simulink model "SimulinkBolaPrato"  (R2020a)
settings: Solver=VariableStepAuto  StartTime=0.0  StopTime=inf  RelTol=1e-3
values from neighbouring files (symbols this model uses):
  A = [0 1;0 -fc/(J/Raio^2+m)]    [TCCMATLAB.m]
  B = [0;-m*g*d/(L*(J/Raio^2+m))]    [TCCMATLAB.m]
  C = [1 0]    [TCCMATLAB.m]
  d = 0.03    [TCCMATLAB.m]
  Kbar = Nu + Klqr*Nx    [TCCMATLAB.m]
  Ki = -K(3)    [TCCMATLAB.m]
  Klqr = lqr(A,B,Q,R)    [TCCMATLAB.m]
  Kt = [K(1) K(2)]    [TCCMATLAB.m]
  L = 1.3    [TCCMATLAB.m]
  Raio = 0.05    [TCCMATLAB.m]
  x0 = 0    [TCCMATLAB.m]
libraries: vrlib x7
settings Model: EnablePacing=on  Creator=Diego  LastModifiedBy=Diego

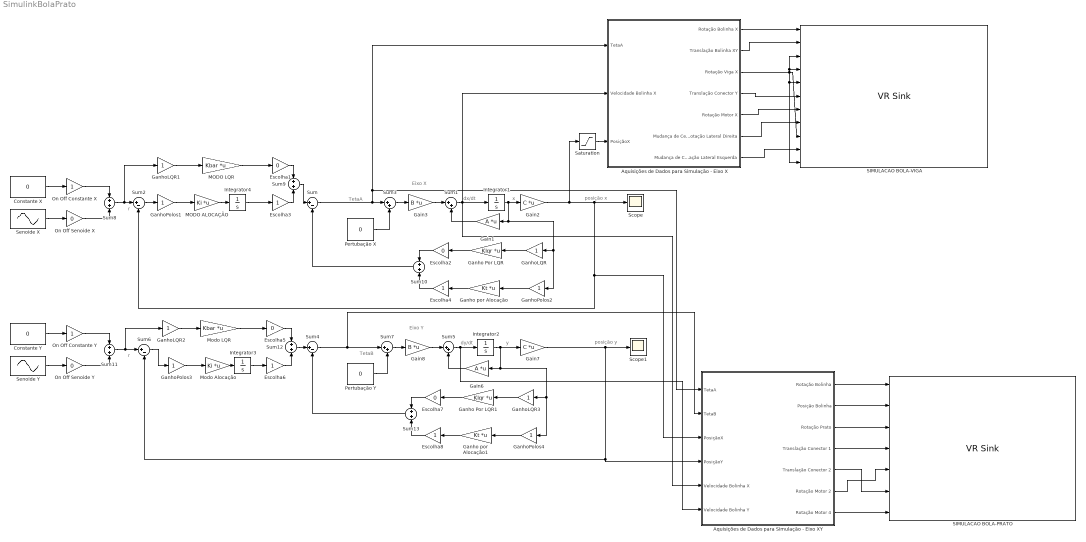
== system SimulinkBolaPrato ==
  note: r
  note: x
  note: posição x
  note: dx/dt
  note: TetaA
  note: Eixo X
  note: TetaB
  note: posição y
  note: dy/dt
  note: y
  note: Eixo Y
  note: r
  Aquisições de Dados para Simulação - Eixo X : Subsystem
  Aquisições de Dados para Simulação - Eixo XY : Subsystem
  Constante X : Constant  Value=0
  Constante Y : Constant  Value=0
  Escolha{1..2,5,7} (4 alike) : Gain  Gain=0
  Escolha{3..4,6,8} (4 alike) : Gain
  Gain1 : Gain  Gain=A  Multiplication=Matrix(K*u)
  Gain2 : Gain  Gain=C  Multiplication=Matrix(K*u)
  Gain3 : Gain  Gain=B  Multiplication=Matrix(K*u)
  Gain6 : Gain  Gain=A  Multiplication=Matrix(K*u)
  Gain7 : Gain  Gain=C  Multiplication=Matrix(K*u)
  Gain8 : Gain  Gain=B  Multiplication=Matrix(K*u)
  Ganho Por LQR : Gain  Gain=Klqr  Multiplication=Matrix(K*u)
  Ganho Por LQR1 : Gain  Gain=Klqr  Multiplication=Matrix(K*u)
  Ganho por Alocação : Gain  Gain=Kt  Multiplication=Matrix(K*u)
  Ganho por Alocação1 : Gain  Gain=Kt  Multiplication=Matrix(K*u)
  GanhoLQR{,1..3} (4 alike) : Gain
  GanhoPolos{1..4} (4 alike) : Gain
  Integrator1 : Integrator  InitialCondition=x0
  Integrator2 : Integrator  InitialCondition=x0
  Integrator3 : Integrator  InitialCondition=x0  AbsoluteTolerance=1
  Integrator4 : Integrator  InitialCondition=x0  AbsoluteTolerance=1
  MODO ALOCAÇÃO : Gain  Gain=Ki  Multiplication=Matrix(K*u)
  MODO LQR : Gain  Gain=Kbar  Multiplication=Matrix(K*u)
  Modo Alocação : Gain  Gain=Ki  Multiplication=Matrix(K*u)
  Modo LQR : Gain  Gain=Kbar  Multiplication=Matrix(K*u)
  On Off Constante X : Gain
  On Off Constante Y : Gain
  On Off Senoide X : Gain  Gain=0
  On Off Senoide Y : Gain  Gain=0
  Pertubação X : Constant  Value=0
  Pertubação Y : Constant  Value=0
  SIMULACAO BOLA-PRATO : vrlib/VR Sink  InstantiateOnLoad=on  SampleTime=-1  ViewEnable=on  RemoteChange=off  RemoteView=off  FieldsWritten=Ball.rotation.4.1.1.double#Ball.translation.3.1.1.double#BaseViga.rotation.4.1.1.double#Conector.translation.3.1.1.double#Motor2.rotation.4.1.1.double#Conector2.translation.3.1.1.double#Motor4.rotation.4.1.1.double  WorldFileName=Ball&Plate.x3d  WorldDescription=Simulação Bola-Prato  AutoView=off  VideoDimensions=[]  AllowVariableSize=off
  SIMULACAO BOLA-VIGA : vrlib/VR Sink  InstantiateOnLoad=on  SampleTime=0.01  ViewEnable=on  RemoteChange=off  RemoteView=off  FieldsWritten=Ball.rotation.4.1.1.double#Ball.translation.3.1.1.double#BaseViga.rotation.4.1.1.double#LadoTraseiroViga.rotation.4.1.1.double#LadoFrontalViga.rotation.4.1.1.double#Conector.translation.3.1.1.double#Motor2.rotation.4.1.1.double#LadoDireitoViga.center.3.1.1.double#LadoDireitoViga.rotation.4.1.1.double#LadoEsquerdoViga.center.3.1.1.double#LadoEsquerdoViga.rotation.4.1.1.double  WorldFileName=Ball&Beam.x3d  AutoView=off  VideoDimensions=[]  AllowVariableSize=off
  Saturation : Saturate  UpperLimit=0.59  LowerLimit=-0.59
  Scope : Scope
  Scope1 : Scope
  Senoide X : Sin  Amplitude=0  SampleTime=0
  Senoide Y : Sin  Amplitude=0  SampleTime=0
  Sum{,2,4,6} (4 alike) : Sum  Inputs=|+-
  Sum{1,3,5,7} (4 alike) : Sum  Inputs=|++
  Sum{8..13} (6 alike) : Sum  Inputs=+|+
  wires:
  Gain3/1 -> Sum1/1
  Gain1/1 -> Sum1/2
  Sum3/1 -> Gain3/1
  MODO ALOCAÇÃO/1 -> Integrator4/1
  Ganho por Alocação/1 -> Escolha4/1
  Sum10/1 -> Sum/2
  Ganho Por LQR/1 -> Escolha2/1
  Senoide X/1 -> On Off Senoide X/1
  Integrator4/1 -> Escolha3/1
  Sum9/1 -> Sum/1
  MODO LQR/1 -> Escolha1/1
  Gain6/1 -> Sum5/2
  Gain8/1 -> Sum5/1
  Sum5/1 -> Aquisições de Dados para Simulação - Eixo XY/6(Velocidade Bolinha Y), Integrator2/1
  Sum7/1 -> Gain8/1
  Integrator2/1 -> GanhoPolos4/1, GanhoLQR3/1, Gain6/1, Gain7/1
  Sum11/1 -> GanhoLQR2/1, Sum6/1
  Gain7/1 -> Sum6/2, Aquisições de Dados para Simulação - Eixo XY/4(PosiçãoY), Scope1/1
  Integrator1/1 -> Gain2/1, GanhoPolos2/1, GanhoLQR/1, Gain1/1
  Gain2/1 -> Saturation/1, Aquisições de Dados para Simulação - Eixo XY/3(PosiçãoX), Sum2/2, Scope/1
  Sum1/1 -> Aquisições de Dados para Simulação - Eixo XY/5(Velocidade Bolinha X), Aquisições de Dados para Simulação - Eixo X/2(Velocidade Bolinha X), Integrator1/1
  Aquisições de Dados para Simulação - Eixo X/1(Rotação Bolinha X) -> SIMULACAO BOLA-VIGA/1
  Aquisições de Dados para Simulação - Eixo X/3(Rotação Viga X) -> SIMULACAO BOLA-VIGA/11, SIMULACAO BOLA-VIGA/5, SIMULACAO BOLA-VIGA/3, SIMULACAO BOLA-VIGA/4, SIMULACAO BOLA-VIGA/9
  Aquisições de Dados para Simulação - Eixo X/2(Translação Bolinha XY) -> SIMULACAO BOLA-VIGA/2
  Aquisições de Dados para Simulação - Eixo X/7(Mudança de Centro de Rotação Lateral Esquerda) -> SIMULACAO BOLA-VIGA/10
  Aquisições de Dados para Simulação - Eixo X/6(Mudança de Centro de Rotação Lateral Direita) -> SIMULACAO BOLA-VIGA/8
  Aquisições de Dados para Simulação - Eixo X/5(Rotação Motor X) -> SIMULACAO BOLA-VIGA/7
  Aquisições de Dados para Simulação - Eixo X/4(Translação Conector Y) -> SIMULACAO BOLA-VIGA/6
  Sum4/1 -> Sum7/1, Aquisições de Dados para Simulação - Eixo XY/2(TetaB)
  Sum/1 -> Aquisições de Dados para Simulação - Eixo XY/1(TetaA), Aquisições de Dados para Simulação - Eixo X/1(TetaA), Sum3/1
  Constante X/1 -> On Off Constante X/1
  Aquisições de Dados para Simulação - Eixo XY/1(Rotação Bolinha) -> SIMULACAO BOLA-PRATO/1
  Aquisições de Dados para Simulação - Eixo XY/2(Posição Bolinha) -> SIMULACAO BOLA-PRATO/2
  Aquisições de Dados para Simulação - Eixo XY/3(Rotação Prato) -> SIMULACAO BOLA-PRATO/3
  Aquisições de Dados para Simulação - Eixo XY/4(Translação Conector 1) -> SIMULACAO BOLA-PRATO/4
  Aquisições de Dados para Simulação - Eixo XY/6(Rotação Motor 2) -> SIMULACAO BOLA-PRATO/5
  Aquisições de Dados para Simulação - Eixo XY/5(Translação Conector 2) -> SIMULACAO BOLA-PRATO/6
  Aquisições de Dados para Simulação - Eixo XY/7(Rotação Motor 4) -> SIMULACAO BOLA-PRATO/7
  Saturation/1 -> Aquisições de Dados para Simulação - Eixo X/3(PosiçãoX)
  Sum8/1 -> GanhoLQR1/1, Sum2/1
  On Off Constante X/1 -> Sum8/1
  On Off Senoide X/1 -> Sum8/2
  Pertubação X/1 -> Sum3/2
  Escolha1/1 -> Sum9/1
  Escolha3/1 -> Sum9/2
  Escolha2/1 -> Sum10/1
  Escolha4/1 -> Sum10/2
  GanhoLQR1/1 -> MODO LQR/1
  GanhoPolos1/1 -> MODO ALOCAÇÃO/1
  Sum2/1 -> GanhoPolos1/1
  GanhoPolos2/1 -> Ganho por Alocação/1
  GanhoLQR/1 -> Ganho Por LQR/1
  Constante Y/1 -> On Off Constante Y/1
  On Off Senoide Y/1 -> Sum11/2
  On Off Constante Y/1 -> Sum11/1
  Modo LQR/1 -> Escolha5/1
  Modo Alocação/1 -> Integrator3/1
  GanhoPolos3/1 -> Modo Alocação/1
  Integrator3/1 -> Escolha6/1
  GanhoLQR2/1 -> Modo LQR/1
  Escolha6/1 -> Sum12/2
  Escolha5/1 -> Sum12/1
  Sum12/1 -> Sum4/1
  Sum6/1 -> GanhoPolos3/1
  Ganho Por LQR1/1 -> Escolha7/1
  Sum13/1 -> Sum4/2
  Ganho por Alocação1/1 -> Escolha8/1
  Escolha7/1 -> Sum13/1
  Escolha8/1 -> Sum13/2
  GanhoLQR3/1 -> Ganho Por LQR1/1
  GanhoPolos4/1 -> Ganho por Alocação1/1
  Pertubação Y/1 -> Sum7/2
  Senoide Y/1 -> On Off Senoide Y/1

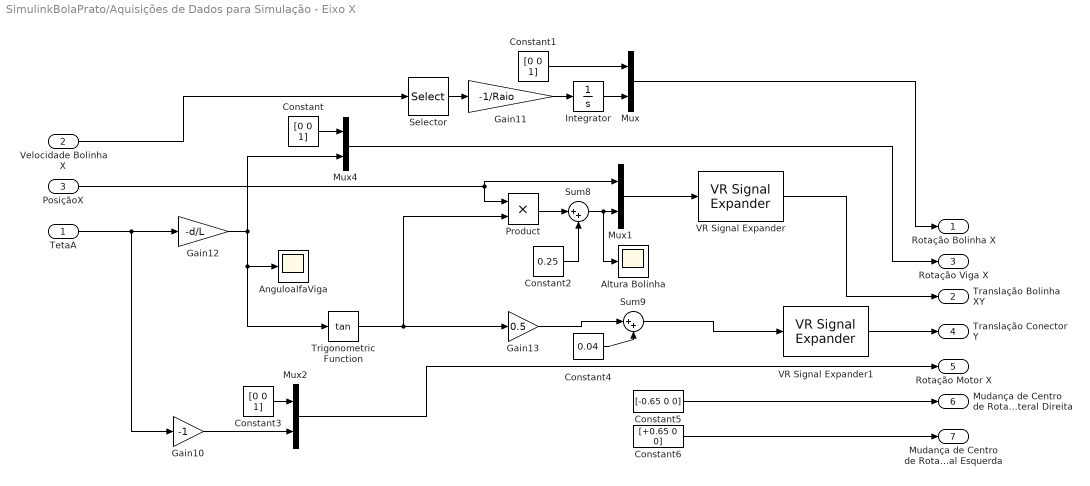
== system SimulinkBolaPrato/Aquisições de Dados para Simulação - Eixo X ==
  TetaA : Inport
  Velocidade Bolinha X : Inport  Port=2
  PosiçãoX : Inport  Port=3
  Altura Bolinha : Scope
  AnguloalfaViga : Scope
  Constant : Constant  Value=[0 0 1]
  Constant1 : Constant  Value=[0 0 1]
  Constant2 : Constant  Value=0.25
  Constant3 : Constant  Value=[0 0 1]
  Constant4 : Constant  Value=0.04
  Constant5 : Constant  Value=[-0.65 0 0]
  Constant6 : Constant  Value=[+0.65 0 0]
  Gain10 : Gain  Gain=-1
  Gain11 : Gain  Gain=-1/Raio
  Gain12 : Gain  Gain=-d/L
  Gain13 : Gain  Gain=0.5
  Integrator : Integrator
  Mux{,1..2,4} (4 alike) : Mux  Inputs=2
  Product : Product
  Selector : Selector  InputPortWidth=2  IndexOptions=Index vector (dialog)  Indices=[1]  OutputSizes=1
  Sum8 : Sum  Inputs=|++
  Sum9 : Sum  Inputs=|++
  Trigonometric Function : Trigonometry  Operator=tan
  VR Signal Expander : vrlib/VR Signal Expander  outwidth=3  outidx=[1 2]
  VR Signal Expander1 : vrlib/VR Signal Expander  outwidth=3  outidx=[2]
  Rotação Bolinha X : Outport
  Translação Bolinha XY : Outport  Port=2
  Rotação Viga X : Outport  Port=3
  Translação Conector Y : Outport  Port=4
  Rotação Motor X : Outport  Port=5
  Mudança de Centro de Rotação Lateral Direita : Outport  Port=6
  Mudança de Centro de Rotação Lateral Esquerda : Outport  Port=7
  wires:
  Constant3/1 -> Mux2/1
  Sum8/1 -> Altura Bolinha/1, Mux1/2
  PosiçãoX/1 -> Product/1, Mux1/1
  Gain13/1 -> Sum9/1
  Sum9/1 -> VR Signal Expander1/1
  Gain10/1 -> Mux2/2
  Constant4/1 -> Sum9/2
  Product/1 -> Sum8/1
  Trigonometric Function/1 -> Product/2, Gain13/1
  Gain12/1 -> Trigonometric Function/1, AnguloalfaViga/1, Mux4/2
  VR Signal Expander1/1 -> Translação Conector Y/1
  TetaA/1 -> Gain10/1, Gain12/1
  Constant2/1 -> Sum8/2
  Constant/1 -> Mux4/1
  Mux1/1 -> VR Signal Expander/1
  Mux2/1 -> Rotação Motor X/1
  Constant5/1 -> Mudança de Centro de Rotação Lateral Direita/1
  Mux4/1 -> Rotação Viga X/1
  Constant6/1 -> Mudança de Centro de Rotação Lateral Esquerda/1
  VR Signal Expander/1 -> Translação Bolinha XY/1
  Velocidade Bolinha X/1 -> Selector/1
  Constant1/1 -> Mux/1
  Gain11/1 -> Integrator/1
  Selector/1 -> Gain11/1
  Mux/1 -> Rotação Bolinha X/1
  Integrator/1 -> Mux/2

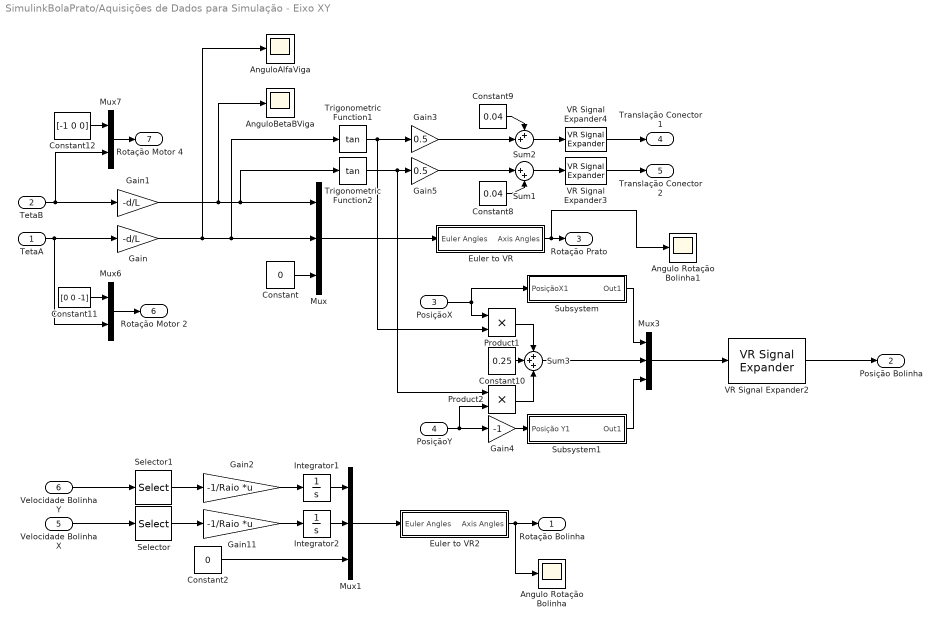
== system SimulinkBolaPrato/Aquisições de Dados para Simulação - Eixo XY ==
  TetaA : Inport
  TetaB : Inport  Port=2
  PosiçãoX : Inport  Port=3
  PosiçãoY : Inport  Port=4
  Velocidade Bolinha X : Inport  Port=5
  Velocidade Bolinha Y : Inport  Port=6
  Angulo Rotação Bolinha : Scope
  Angulo Rotação Bolinha1 : Scope
  AnguloAlfaViga : Scope
  AnguloBetaBViga : Scope
  Constant : Constant  Value=0
  Constant10 : Constant  Value=0.25
  Constant11 : Constant  Value=[0 0 -1]
  Constant12 : Constant  Value=[-1 0 0]
  Constant2 : Constant  Value=0
  Constant8 : Constant  Value=0.04
  Constant9 : Constant  Value=0.04
  Euler to VR : Subsystem
  Euler to VR2 : Subsystem
  Gain : Gain  Gain=-d/L
  Gain1 : Gain  Gain=-d/L
  Gain11 : Gain  Gain=-1/Raio  Multiplication=Matrix(K*u)
  Gain2 : Gain  Gain=-1/Raio  Multiplication=Matrix(K*u)
  Gain3 : Gain  Gain=0.5
  Gain4 : Gain  Gain=-1
  Gain5 : Gain  Gain=0.5
  Integrator1 : Integrator
  Integrator2 : Integrator
  Mux : Mux  Inputs=3
  Mux1 : Mux  Inputs=3
  Mux3 : Mux  Inputs=3
  Mux6 : Mux  Inputs=2
  Mux7 : Mux  Inputs=2
  Product1 : Product
  Product2 : Product
  Selector : Selector  InputPortWidth=2  IndexOptions=Index vector (dialog)  Indices=[1]  OutputSizes=1
  Selector1 : Selector  InputPortWidth=2  IndexOptions=Index vector (dialog)  Indices=[1]  OutputSizes=1
  Subsystem : Subsystem
  Subsystem1 : Subsystem
  Sum1 : Sum  Inputs=|++
  Sum2 : Sum  Inputs=++|
  Sum3 : Sum  Inputs=+++
  Trigonometric Function1 : Trigonometry  Operator=tan
  Trigonometric Function2 : Trigonometry  Operator=tan
  VR Signal Expander2 : vrlib/VR Signal Expander  outwidth=3  outidx=[1 2 3]
  VR Signal Expander3 : vrlib/VR Signal Expander  outwidth=3  outidx=[2]
  VR Signal Expander4 : vrlib/VR Signal Expander  outwidth=3  outidx=[2]
  Rotação Bolinha : Outport
  Posição Bolinha : Outport  Port=2
  Rotação Prato : Outport  Port=3
  Translação Conector 1 : Outport  Port=4
  Translação Conector 2 : Outport  Port=5
  Rotação Motor 2 : Outport  Port=6
  Rotação Motor 4 : Outport  Port=7
  wires:
  Mux/1 -> Euler to VR/1(Euler Angles)
  Constant/1 -> Mux/3
  Gain/1 -> AnguloAlfaViga/1, Trigonometric Function1/1, Mux/2
  Gain1/1 -> AnguloBetaBViga/1, Mux/1, Trigonometric Function2/1
  TetaB/1 -> Gain1/1, Mux7/2
  Mux3/1 -> VR Signal Expander2/1
  Selector1/1 -> Gain2/1
  Velocidade Bolinha Y/1 -> Selector1/1
  Mux1/1 -> Euler to VR2/1(Euler Angles)
  Constant2/1 -> Mux1/3
  PosiçãoY/1 -> Product2/2, Gain4/1
  VR Signal Expander2/1 -> Posição Bolinha/1
  Euler to VR/1(Axis Angles) -> Angulo Rotação Bolinha1/1, Rotação Prato/1
  Trigonometric Function1/1 -> Product1/2, Gain3/1
  Trigonometric Function2/1 -> Product2/1, Gain5/1
  VR Signal Expander3/1 -> Translação Conector 2/1
  Constant8/1 -> Sum1/2
  Sum1/1 -> VR Signal Expander3/1
  Gain5/1 -> Sum1/1
  VR Signal Expander4/1 -> Translação Conector 1/1
  Sum2/1 -> VR Signal Expander4/1
  Gain3/1 -> Sum2/2
  Constant9/1 -> Sum2/1
  Selector/1 -> Gain11/1
  Velocidade Bolinha X/1 -> Selector/1
  Product1/1 -> Sum3/1
  Product2/1 -> Sum3/3
  Constant10/1 -> Sum3/2
  Sum3/1 -> Mux3/2
  TetaA/1 -> Gain/1, Mux6/2
  Constant11/1 -> Mux6/1
  Mux6/1 -> Rotação Motor 2/1
  Mux7/1 -> Rotação Motor 4/1
  Constant12/1 -> Mux7/1
  PosiçãoX/1 -> Subsystem/1(PosiçãoX1), Product1/1
  Subsystem/1(Out1) -> Mux3/1
  Gain4/1 -> Subsystem1/1(Posição Y1)
  Subsystem1/1(Out1) -> Mux3/3
  Gain2/1 -> Integrator1/1
  Gain11/1 -> Integrator2/1
  Euler to VR2/1(Axis Angles) -> Rotação Bolinha/1, Angulo Rotação Bolinha/1
  Integrator1/1 -> Mux1/1
  Integrator2/1 -> Mux1/2

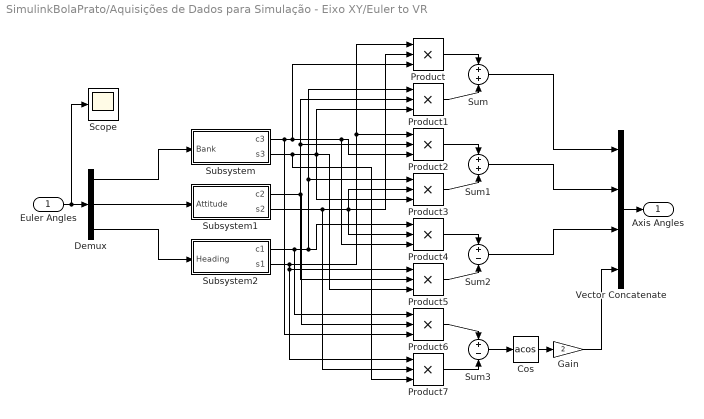
== system SimulinkBolaPrato/Aquisições de Dados para Simulação - Eixo XY/Euler to VR ==
  Euler Angles : Inport
  Cos : Trigonometry  Operator=acos
  Demux : Demux  Outputs=3
      settings: DisplayOption=none
  Gain : Gain  Gain=2
  Product{,1..7} (8 alike) : Product  Inputs=3
  Scope : Scope
  Subsystem : Subsystem
  Subsystem1 : Subsystem
  Subsystem2 : Subsystem
  Sum : Sum  Inputs=+|+
  Sum1 : Sum  Inputs=+|+
  Sum2 : Sum  Inputs=+|-
  Sum3 : Sum  Inputs=+|-
  Vector Concatenate : Concatenate  NumInputs=4
  Axis Angles : Outport
  wires:
  Euler Angles/1 -> Scope/1, Demux/1
  Demux/1 -> Subsystem/1(Bank)
  Demux/3 -> Subsystem2/1(Heading)
  Demux/2 -> Subsystem1/1(Attitude)
  Subsystem2/2(s1) -> Product7/1, Product5/1, Product2/1, Product/1
  Subsystem1/2(s2) -> Product7/2, Product3/2, Product/2, Product4/2
  Subsystem/1(c3) -> Product6/3, Product4/3, Product2/3, Product/3
  Subsystem2/1(c1) -> Product6/1, Product4/1, Product3/1, Product1/1
  Subsystem1/1(c2) -> Product6/2, Product5/2, Product2/2, Product1/2
  Subsystem/2(s3) -> Product7/3, Product5/3, Product1/3, Product3/3
  Product/1 -> Sum/1
  Product1/1 -> Sum/2
  Product2/1 -> Sum1/1
  Product3/1 -> Sum1/2
  Product4/1 -> Sum2/1
  Product5/1 -> Sum2/2
  Product6/1 -> Sum3/1
  Product7/1 -> Sum3/2
  Sum3/1 -> Cos/1
  Cos/1 -> Gain/1
  Gain/1 -> Vector Concatenate/4
  Sum/1 -> Vector Concatenate/1
  Sum1/1 -> Vector Concatenate/2
  Sum2/1 -> Vector Concatenate/3
  Vector Concatenate/1 -> Axis Angles/1

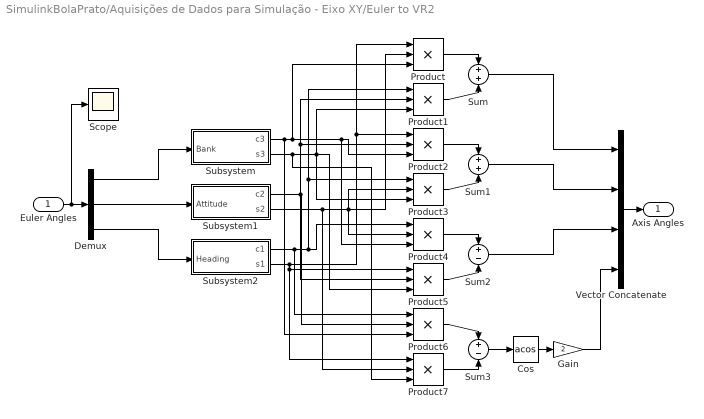
== system SimulinkBolaPrato/Aquisições de Dados para Simulação - Eixo XY/Euler to VR2 ==
  Euler Angles : Inport
  Cos : Trigonometry  Operator=acos
  Demux : Demux  Outputs=3
      settings: DisplayOption=none
  Gain : Gain  Gain=2
  Product{,1..7} (8 alike) : Product  Inputs=3
  Scope : Scope
  Subsystem : Subsystem
  Subsystem1 : Subsystem
  Subsystem2 : Subsystem
  Sum : Sum  Inputs=+|+
  Sum1 : Sum  Inputs=+|+
  Sum2 : Sum  Inputs=+|-
  Sum3 : Sum  Inputs=+|-
  Vector Concatenate : Concatenate  NumInputs=4
  Axis Angles : Outport
  wires:
  Euler Angles/1 -> Scope/1, Demux/1
  Demux/1 -> Subsystem/1(Bank)
  Demux/3 -> Subsystem2/1(Heading)
  Demux/2 -> Subsystem1/1(Attitude)
  Subsystem2/2(s1) -> Product7/1, Product5/1, Product2/1, Product/1
  Subsystem1/2(s2) -> Product7/2, Product3/2, Product/2, Product4/2
  Subsystem/1(c3) -> Product6/3, Product4/3, Product2/3, Product/3
  Subsystem2/1(c1) -> Product6/1, Product4/1, Product3/1, Product1/1
  Subsystem1/1(c2) -> Product6/2, Product5/2, Product2/2, Product1/2
  Subsystem/2(s3) -> Product7/3, Product5/3, Product1/3, Product3/3
  Product/1 -> Sum/1
  Product1/1 -> Sum/2
  Product2/1 -> Sum1/1
  Product3/1 -> Sum1/2
  Product4/1 -> Sum2/1
  Product5/1 -> Sum2/2
  Product6/1 -> Sum3/1
  Product7/1 -> Sum3/2
  Sum3/1 -> Cos/1
  Cos/1 -> Gain/1
  Vector Concatenate/1 -> Axis Angles/1
  Sum/1 -> Vector Concatenate/1
  Sum2/1 -> Vector Concatenate/3
  Sum1/1 -> Vector Concatenate/2
  Gain/1 -> Vector Concatenate/4

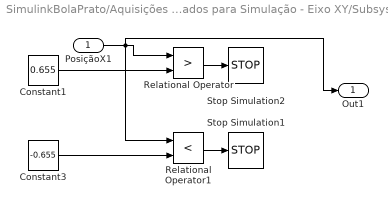
== system SimulinkBolaPrato/Aquisições de Dados para Simulação - Eixo XY/Subsystem ==
  PosiçãoX1 : Inport
  Constant1 : Constant  Value=0.655
  Constant3 : Constant  Value=-0.655
  Relational Operator : RelationalOperator  Operator=>  OutDataTypeStr=boolean  RndMeth=Simplest
  Relational Operator1 : RelationalOperator  Operator=<  OutDataTypeStr=boolean  RndMeth=Simplest
  Stop Simulation1 : Stop
  Stop Simulation2 : Stop
  Out1 : Outport
  wires:
  Constant1/1 -> Relational Operator/2
  PosiçãoX1/1 -> Relational Operator1/1, Out1/1, Relational Operator/1
  Relational Operator/1 -> Stop Simulation2/1
  Relational Operator1/1 -> Stop Simulation1/1
  Constant3/1 -> Relational Operator1/2

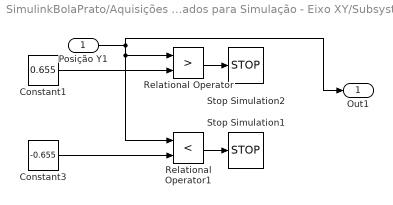
== system SimulinkBolaPrato/Aquisições de Dados para Simulação - Eixo XY/Subsystem1 ==
  Posição Y1 : Inport
  Constant1 : Constant  Value=0.655
  Constant3 : Constant  Value=-0.655
  Relational Operator : RelationalOperator  Operator=>  OutDataTypeStr=boolean  RndMeth=Simplest
  Relational Operator1 : RelationalOperator  Operator=<  OutDataTypeStr=boolean  RndMeth=Simplest
  Stop Simulation1 : Stop
  Stop Simulation2 : Stop
  Out1 : Outport
  wires:
  Relational Operator/1 -> Stop Simulation2/1
  Constant3/1 -> Relational Operator1/2
  Relational Operator1/1 -> Stop Simulation1/1
  Constant1/1 -> Relational Operator/2
  Posição Y1/1 -> Relational Operator1/1, Relational Operator/1, Out1/1

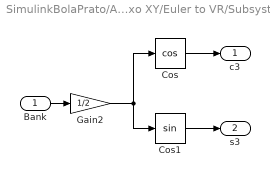
== system SimulinkBolaPrato/Aquisições de Dados para Simulação - Eixo XY/Euler to VR/Subsystem ==
  Bank : Inport
  Cos : Trigonometry  Operator=cos
  Cos1 : Trigonometry
  Gain2 : Gain  Gain=1/2
  c3 : Outport
  s3 : Outport  Port=2
  wires:
  Cos/1 -> c3/1
  Gain2/1 -> Cos/1, Cos1/1
  Bank/1 -> Gain2/1
  Cos1/1 -> s3/1

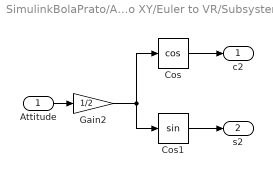
== system SimulinkBolaPrato/Aquisições de Dados para Simulação - Eixo XY/Euler to VR/Subsystem1 ==
  Attitude : Inport
  Cos : Trigonometry  Operator=cos
  Cos1 : Trigonometry
  Gain2 : Gain  Gain=1/2
  c2 : Outport
  s2 : Outport  Port=2
  wires:
  Cos/1 -> c2/1
  Gain2/1 -> Cos/1, Cos1/1
  Attitude/1 -> Gain2/1
  Cos1/1 -> s2/1

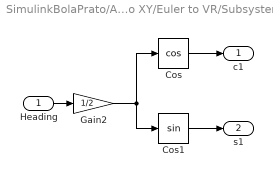
== system SimulinkBolaPrato/Aquisições de Dados para Simulação - Eixo XY/Euler to VR/Subsystem2 ==
  Heading : Inport
  Cos : Trigonometry  Operator=cos
  Cos1 : Trigonometry
  Gain2 : Gain  Gain=1/2
  c1 : Outport
  s1 : Outport  Port=2
  wires:
  Cos/1 -> c1/1
  Gain2/1 -> Cos/1, Cos1/1
  Heading/1 -> Gain2/1
  Cos1/1 -> s1/1

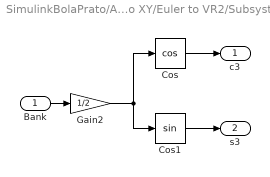
== system SimulinkBolaPrato/Aquisições de Dados para Simulação - Eixo XY/Euler to VR2/Subsystem ==
  Bank : Inport
  Cos : Trigonometry  Operator=cos
  Cos1 : Trigonometry
  Gain2 : Gain  Gain=1/2
  c3 : Outport
  s3 : Outport  Port=2
  wires:
  Cos/1 -> c3/1
  Gain2/1 -> Cos/1, Cos1/1
  Bank/1 -> Gain2/1
  Cos1/1 -> s3/1

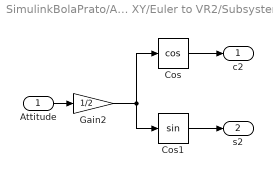
== system SimulinkBolaPrato/Aquisições de Dados para Simulação - Eixo XY/Euler to VR2/Subsystem1 ==
  Attitude : Inport
  Cos : Trigonometry  Operator=cos
  Cos1 : Trigonometry
  Gain2 : Gain  Gain=1/2
  c2 : Outport
  s2 : Outport  Port=2
  wires:
  Cos/1 -> c2/1
  Gain2/1 -> Cos/1, Cos1/1
  Attitude/1 -> Gain2/1
  Cos1/1 -> s2/1

== system SimulinkBolaPrato/Aquisições de Dados para Simulação - Eixo XY/Euler to VR2/Subsystem2 ==
  Heading : Inport
  Cos : Trigonometry  Operator=cos
  Cos1 : Trigonometry
  Gain2 : Gain  Gain=1/2
  c1 : Outport
  s1 : Outport  Port=2
  wires:
  Cos/1 -> c1/1
  Gain2/1 -> Cos/1, Cos1/1
  Heading/1 -> Gain2/1
  Cos1/1 -> s1/1
